simulink model "sf_tictacflow"  (Simulink 7.6)
settings: Solver=VariableStepDiscrete  StartTime=0.0  StopTime=inf  RelTol=1e-3
settings Model: Creator=The MathWorks Inc.  CovMetricSettings=dcmtr  ExtModeTrigMode=oneshot  ExtModeArmWhenConnect=off  ExtModeAutoUpdateStatusClock=off
settings DataIOCC: LimitDataPoints=off  SaveOutput=off  SaveTime=off  SignalLoggingName=sigsOut
settings OptimizationCC: BlockReduction=off  BooleanDataType=off  InlineInvariantSignals=on  InitFltsAndDblsToZero=on  EfficientMapNaN2IntZero=off  BufferReusableBoundary=off
settings DebuggingCC: SaveWithParameterizedLinksMsg=none  SignalResolutionControl=TryResolveAllWithWarning  SolverPrmCheckMsg=none  MultiTaskDSMMsg=warning  MultiTaskCondExecSysMsg=none  BusObjectLabelMismatch=none  StrictBusMsg=None
settings HardwareCC: TargetUnknown=on
settings SFSimCC: SFSimEcho=off  SimParseCustomCode=off
settings RTWCC: IncludeERTFirstTime=on
settings GRTTargetCC: TargetFcnLib=ansi_tfl_tmw.mat

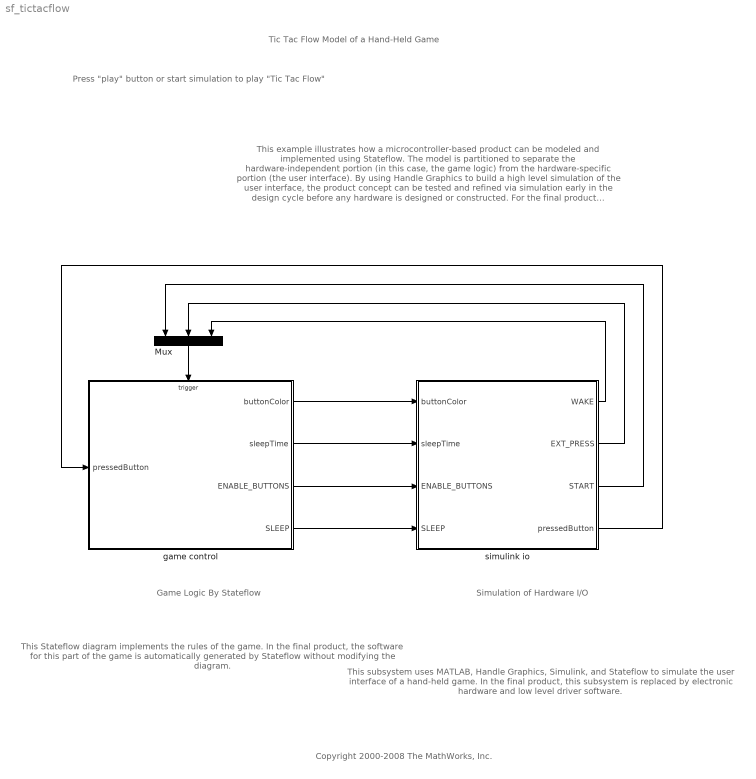
== system sf_tictacflow ==
  note: Press "play" button or start simulation to play "Tic Tac Flow"
  note: This Stateflow diagram implements
      | the rules of the game.
      |
      | In the final product, the software for this
      | part of the game is automatically generated
      |  by Stateflow without modifying the diagram.
  note: Game Logic By Stateflow
  note: This subsystem uses MATLAB, Handle
      | Graphics, Simulink, and Stateflow
      |  to simulate the user interface of a
      | hand-held game.
      |
      | In the final product, this subsystem is
      | replaced by electronic hardware and
      | low level driver software.
  note: This example illustrates how a microcontroller-based product can be modeled and implemented using Stateflow.
      |
      | The model is partitioned to separate the hardware-independent portion (in
      | this case, the game logic) from the hardware-specific portion (the user interface).
      | By using Handle Graphics to build a high level simulation of the user interface, the product concept can
      |  be tested and refined via simulation early in the design cycle before any hardware is designed or constructed.
      | For the final product implementation, the hardware-independent portion is implemented automatically
      |  by Stateflow, while the hardware-specific portion is replaced by actual hardware and low-level driver software.
  note: Tic Tac Flow
      | Model of a Hand-Held Game
  note: Simulation of Hardware I/O
  note: Copyright 2000-2008 The MathWorks, Inc.
  Mux : Mux  Inputs=3
  game control : Stateflow chart  TreatAsAtomicUnit=on
  simulink io : Subsystem  StopFcn=if ishandle(1.000000); delete(1.000000); end;
  wires:
  Mux/1 -> game control/Trigger
  game control/2(sleepTime) -> simulink io/2(sleepTime)
  game control/3(ENABLE_BUTTONS) -> simulink io/3(ENABLE_BUTTONS)
  game control/4(SLEEP) -> simulink io/4(SLEEP)
  game control/1(buttonColor) -> simulink io/1(buttonColor)
  simulink io/1(WAKE) -> Mux/3
  simulink io/2(EXT_PRESS) -> Mux/2
  simulink io/3(START) -> Mux/1
  simulink io/4(pressedButton) -> game control/1(pressedButton)

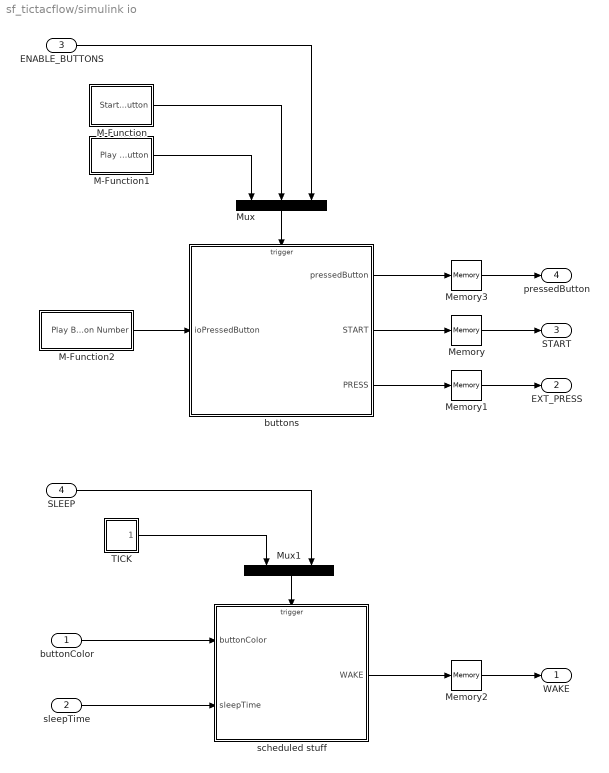
== system sf_tictacflow/simulink io ==
  buttonColor : Inport
  sleepTime : Inport  Port=2
  ENABLE_BUTTONS : Inport  Port=3
  SLEEP : Inport  Port=4
  M-Function : Subsystem
  M-Function1 : Subsystem
  M-Function2 : Subsystem
  Memory{,1..3} (4 alike) : Memory
  Mux : Mux  Inputs=3
  Mux1 : Mux  Inputs=2
  TICK : Subsystem  mask(Pulse Generator){period=1/60, duty=50, amplitude=1, start=0}
      mask prompts: period "Period (secs):"; duty "Duty cycle (% of period):"; start "Start time:"
      mask help: Pulse Generator
      mask Help: Pulse generator which ensures pulse transitions are hit. Provides a vector of pulses when the height is entered as a vector.  Unmask to see how it works.
      mask Display: plot(0,0,100,100,[95,90,90,75,75,60,60,45,45,30,30,15,15,5],[25,25,75,75,25,25,75,75,25,25,75,75,25,25]);
  buttons : Stateflow chart  TreatAsAtomicUnit=on
  scheduled stuff : Stateflow chart  TreatAsAtomicUnit=on
  WAKE : Outport
  EXT_PRESS : Outport  Port=2
  START : Outport  Port=3
  pressedButton : Outport  Port=4
  wires:
  Mux/1 -> buttons/Trigger
  Mux1/1 -> scheduled stuff/Trigger
  scheduled stuff/1(WAKE) -> Memory2/1
  Memory2/1 -> WAKE/1
  sleepTime/1 -> scheduled stuff/2(sleepTime)
  buttonColor/1 -> scheduled stuff/1(buttonColor)
  TICK/1(Out1) -> Mux1/1
  SLEEP/1 -> Mux1/2
  M-Function2/1(Play Button Number) -> buttons/1(ioPressedButton)
  M-Function1/1(Play Button) -> Mux/1
  M-Function/1(Start Button) -> Mux/2
  ENABLE_BUTTONS/1 -> Mux/3
  buttons/1(pressedButton) -> Memory3/1
  buttons/2(START) -> Memory/1
  Memory/1 -> START/1
  buttons/3(PRESS) -> Memory1/1
  Memory1/1 -> EXT_PRESS/1
  Memory3/1 -> pressedButton/1

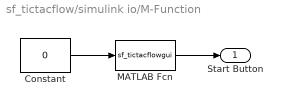
== system sf_tictacflow/simulink io/M-Function ==
  Constant : Constant  Value=0
  MATLAB Fcn : MATLABFcn  MATLABFcn=sf_tictacflowgui
  Start Button : Outport
  wires:
  Constant/1 -> MATLAB Fcn/1
  MATLAB Fcn/1 -> Start Button/1

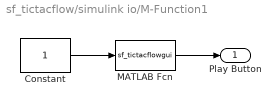
== system sf_tictacflow/simulink io/M-Function1 ==
  Constant : Constant
  MATLAB Fcn : MATLABFcn  MATLABFcn=sf_tictacflowgui
  Play Button : Outport
  wires:
  MATLAB Fcn/1 -> Play Button/1
  Constant/1 -> MATLAB Fcn/1

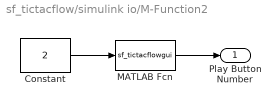
== system sf_tictacflow/simulink io/M-Function2 ==
  Constant : Constant  Value=2
  MATLAB Fcn : MATLABFcn  MATLABFcn=sf_tictacflowgui
  Play Button Number : Outport
  wires:
  Constant/1 -> MATLAB Fcn/1
  MATLAB Fcn/1 -> Play Button Number/1

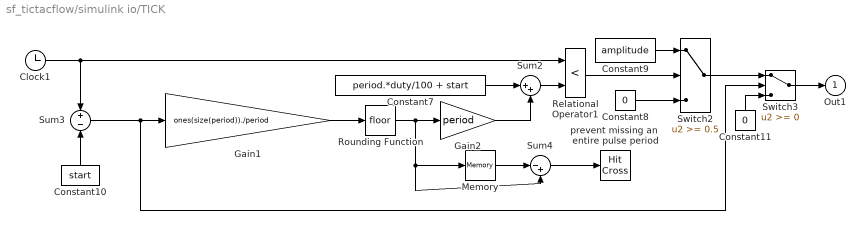
== system sf_tictacflow/simulink io/TICK ==
  Clock1 : Clock
      settings: Decimation=10
  Constant10 : Constant  Value=start
  Constant11 : Constant  Value=0
  Constant7 : Constant  Value=period.*duty/100 + start
  Constant8 : Constant  Value=0
  Constant9 : Constant  Value=amplitude
  Gain1 : Gain  Gain=ones(size(period))./period  SaturateOnIntegerOverflow=on  OutDataTypeStr=Inherit: Same as input  ParamDataTypeStr=Inherit: Same as input
  Gain2 : Gain  Gain=period  SaturateOnIntegerOverflow=on  OutDataTypeStr=Inherit: Same as input  ParamDataTypeStr=Inherit: Same as input
  Memory : Memory
  Relational Operator1 : RelationalOperator  Operator=<  InputSameDT=on
  Rounding Function : Rounding
  Sum2 : Sum  Inputs=|++  SaturateOnIntegerOverflow=on  InputSameDT=on  OutDataTypeStr=Inherit: Same as first input
  Sum3 : Sum  Inputs=+-  SaturateOnIntegerOverflow=on  InputSameDT=on  OutDataTypeStr=Inherit: Same as first input
  Sum4 : Sum  Inputs=|-+  SaturateOnIntegerOverflow=on  InputSameDT=on  OutDataTypeStr=Inherit: Same as first input
  Switch2 : Switch  Threshold=0.5  SaturateOnIntegerOverflow=on  InputSameDT=on
  Switch3 : Switch  SaturateOnIntegerOverflow=on  InputSameDT=on
  prevent missing an  entire pulse period : HitCross  HitCrossingOffset=1  ShowOutputPort=off
  Out1 : Outport
  wires:
  Memory/1 -> Sum4/1
  Sum4/1 -> prevent missing an  entire pulse period/1
  Switch2/1 -> Switch3/1
  Constant11/1 -> Switch3/3
  Constant9/1 -> Switch2/1
  Constant8/1 -> Switch2/3
  Relational Operator1/1 -> Switch2/2
  Switch3/1 -> Out1/1
  Rounding Function/1 -> Gain2/1, Memory/1, Sum4/2
  Gain2/1 -> Sum2/2
  Constant7/1 -> Sum2/1
  Gain1/1 -> Rounding Function/1
  Sum2/1 -> Relational Operator1/2
  Clock1/1 -> Sum3/1, Relational Operator1/1
  Sum3/1 -> Switch3/2, Gain1/1
  Constant10/1 -> Sum3/2

== stateflow chart game control ==
  settings: executeAtInitialization=1
  state button_7 [parallel]
    settings: executionOrder=1
    state enabled
      buttonColor[thisButton] = DARK;
    state active
      state green
        buttonColor[thisButton] = GREEN;
        TURN;
      state red
        buttonColor[thisButton] = RED;
        TURN;
      (junction 82) -> button_7.active.green [order 1] : [in(turn.green)]
      (junction 82) -> button_7.active.red [order 2]
    state disabled
    button_7.active.green -> button_7.disabled : GAME_OVER [in(turn.red)]
        | {buttonColor[thisButton] = DIM_GREEN; }
    button_7.enabled -> button_7.disabled [order 1] : GAME_OVER
    button_7 -> (junction 86) : START
    button_7.active -> button_7.enabled : at(7,TURN)
    (junction 86) -> button_7.enabled
    (default) -> (junction 86)
    button_7.enabled -> (junction 82) [order 2] : PRESS
    button_7.active.red -> button_7.disabled : GAME_OVER [in(turn.green)]
        | {buttonColor[thisButton] = DIM_RED; }
  state button_0 [parallel]
    settings: executionOrder=2
    state disabled
    state enabled
      buttonColor[thisButton] = DARK;
    state active
      state red
        buttonColor[thisButton] = RED;
        TURN;
      state green
        buttonColor[thisButton] = GREEN;
        TURN;
      (junction 105) -> button_0.active.red [order 2]
      (junction 105) -> button_0.active.green [order 1] : [in(turn.green)]
    button_0 -> (junction 104) : START
    (default) -> (junction 104)
    (junction 104) -> button_0.enabled
    button_0.enabled -> button_0.disabled [order 1] : GAME_OVER
    button_0.active.red -> button_0.disabled : GAME_OVER [in(turn.green)]
        | {buttonColor[thisButton] = DIM_RED; }
    button_0.active.green -> button_0.disabled : GAME_OVER [in(turn.red)]
        | {buttonColor[thisButton] = DIM_GREEN; }
    button_0.active -> button_0.enabled : at(7,TURN)
    button_0.enabled -> (junction 105) [order 2] : PRESS
  state button_5 [parallel]
    settings: executionOrder=3
    state disabled
    state enabled
      buttonColor[thisButton] = DARK;
    state active
      state red
        buttonColor[thisButton] = RED;
        TURN;
      state green
        buttonColor[thisButton] = GREEN;
        TURN;
      (junction 107) -> button_5.active.red [order 2]
      (junction 107) -> button_5.active.green [order 1] : [in(turn.green)]
    button_5 -> (junction 106) : START
    (default) -> (junction 106)
    (junction 106) -> button_5.enabled
    button_5.enabled -> button_5.disabled [order 1] : GAME_OVER
    button_5.active.red -> button_5.disabled : GAME_OVER [in(turn.green)]
        | {buttonColor[thisButton] = DIM_RED; }
    button_5.active.green -> button_5.disabled : GAME_OVER [in(turn.red)]
        | {buttonColor[thisButton] = DIM_GREEN; }
    button_5.active -> button_5.enabled : at(7,TURN)
    button_5.enabled -> (junction 107) [order 2] : PRESS
  state button_6 [parallel]
    settings: executionOrder=6
    state disabled
    state enabled
      buttonColor[thisButton] = DARK;
    state active
      state red
        buttonColor[thisButton] = RED;
        TURN;
      state green
        buttonColor[thisButton] = GREEN;
        TURN;
      (junction 109) -> button_6.active.red [order 2]
      (junction 109) -> button_6.active.green [order 1] : [in(turn.green)]
    button_6 -> (junction 108) : START
    (default) -> (junction 108)
    (junction 108) -> button_6.enabled
    button_6.enabled -> button_6.disabled [order 1] : GAME_OVER
    button_6.active.red -> button_6.disabled : GAME_OVER [in(turn.green)]
        | {buttonColor[thisButton] = DIM_RED; }
    button_6.active.green -> button_6.disabled : GAME_OVER [in(turn.red)]
        | {buttonColor[thisButton] = DIM_GREEN; }
    button_6.active -> button_6.enabled : at(7,TURN)
    button_6.enabled -> (junction 109) [order 2] : PRESS
  state button_4 [parallel]
    settings: executionOrder=5
    state disabled
    state enabled
      buttonColor[thisButton] = DARK;
    state active
      state red
        buttonColor[thisButton] = RED;
        TURN;
      state green
        buttonColor[thisButton] = GREEN;
        TURN;
      (junction 111) -> button_4.active.red [order 2]
      (junction 111) -> button_4.active.green [order 1] : [in(turn.green)]
    button_4 -> (junction 110) : START
    (default) -> (junction 110)
    (junction 110) -> button_4.enabled
    button_4.enabled -> button_4.disabled [order 1] : GAME_OVER
    button_4.active.red -> button_4.disabled : GAME_OVER [in(turn.green)]
        | {buttonColor[thisButton] = DIM_RED; }
    button_4.active.green -> button_4.disabled : GAME_OVER [in(turn.red)]
        | {buttonColor[thisButton] = DIM_GREEN; }
    button_4.active -> button_4.enabled : at(7,TURN)
    button_4.enabled -> (junction 111) [order 2] : PRESS
  state button_2 [parallel]
    settings: executionOrder=4
    state disabled
    state enabled
      buttonColor[thisButton] = DARK;
    state active
      state red
        buttonColor[thisButton] = RED;
        TURN;
      state green
        buttonColor[thisButton] = GREEN;
        TURN;
      (junction 113) -> button_2.active.red [order 2]
      (junction 113) -> button_2.active.green [order 1] : [in(turn.green)]
    button_2 -> (junction 112) : START
    (default) -> (junction 112)
    (junction 112) -> button_2.enabled
    button_2.enabled -> button_2.disabled [order 1] : GAME_OVER
    button_2.active.red -> button_2.disabled : GAME_OVER [in(turn.green)]
        | {buttonColor[thisButton] = DIM_RED; }
    button_2.active.green -> button_2.disabled : GAME_OVER [in(turn.red)]
        | {buttonColor[thisButton] = DIM_GREEN; }
    button_2.active -> button_2.enabled : at(7,TURN)
    button_2.enabled -> (junction 113) [order 2] : PRESS
  state button_1 [parallel]
    settings: executionOrder=9
    state disabled
    state enabled
      buttonColor[thisButton] = DARK;
    state active
      state red
        buttonColor[thisButton] = RED;
        TURN;
      state green
        buttonColor[thisButton] = GREEN;
        TURN;
      (junction 115) -> button_1.active.red [order 2]
      (junction 115) -> button_1.active.green [order 1] : [in(turn.green)]
    button_1 -> (junction 114) : START
    (default) -> (junction 114)
    (junction 114) -> button_1.enabled
    button_1.enabled -> button_1.disabled [order 1] : GAME_OVER
    button_1.active.red -> button_1.disabled : GAME_OVER [in(turn.green)]
        | {buttonColor[thisButton] = DIM_RED; }
    button_1.active.green -> button_1.disabled : GAME_OVER [in(turn.red)]
        | {buttonColor[thisButton] = DIM_GREEN; }
    button_1.active -> button_1.enabled : at(7,TURN)
    button_1.enabled -> (junction 115) [order 2] : PRESS
  state button_8 [parallel]
    settings: executionOrder=8
    state disabled
    state enabled
      buttonColor[thisButton] = DARK;
    state active
      state red
        buttonColor[thisButton] = RED;
        TURN;
      state green
        buttonColor[thisButton] = GREEN;
        TURN;
      (junction 117) -> button_8.active.red [order 2]
      (junction 117) -> button_8.active.green [order 1] : [in(turn.green)]
    button_8 -> (junction 116) : START
    (default) -> (junction 116)
    (junction 116) -> button_8.enabled
    button_8.enabled -> button_8.disabled [order 1] : GAME_OVER
    button_8.active.red -> button_8.disabled : GAME_OVER [in(turn.green)]
        | {buttonColor[thisButton] = DIM_RED; }
    button_8.active.green -> button_8.disabled : GAME_OVER [in(turn.red)]
        | {buttonColor[thisButton] = DIM_GREEN; }
    button_8.active -> button_8.enabled : at(7,TURN)
    button_8.enabled -> (junction 117) [order 2] : PRESS
  state button_3 [parallel]
    settings: executionOrder=7
    state disabled
    state enabled
      buttonColor[thisButton] = DARK;
    state active
      state red
        buttonColor[thisButton] = RED;
        TURN;
      state green
        buttonColor[thisButton] = GREEN;
        TURN;
      (junction 119) -> button_3.active.red [order 2]
      (junction 119) -> button_3.active.green [order 1] : [in(turn.green)]
    button_3 -> (junction 118) : START
    (default) -> (junction 118)
    (junction 118) -> button_3.enabled
    button_3.enabled -> button_3.disabled [order 1] : GAME_OVER
    button_3.active.red -> button_3.disabled : GAME_OVER [in(turn.green)]
        | {buttonColor[thisButton] = DIM_RED; }
    button_3.active.green -> button_3.disabled : GAME_OVER [in(turn.red)]
        | {buttonColor[thisButton] = DIM_GREEN; }
    button_3.active -> button_3.enabled : at(7,TURN)
    button_3.enabled -> (junction 119) [order 2] : PRESS
  state turn [parallel]
    settings: executionOrder=10
    state yes = make_move_if_available(move) [function]
      (junction 89) -> (junction 77)
      (junction 97) -> (junction 88) [order 2]
      (junction 88) -> (junction 78) [order 1] : [ move == 8 && in(button_8.enabled)] { shift_game_state(move); send(PRESS,button_8);}
      (junction 99) -> (junction 97) [order 2]
      (default) -> (junction 70)
      (junction 98) -> (junction 96)
      (junction 88) -> (junction 85) [order 2] : { yes = 0; }
      (junction 97) -> (junction 96) [order 1] : [ move == 7 && in(button_7.enabled)] { shift_game_state(move); send(PRESS,button_7);}
      (junction 70) -> (junction 80) [order 1] : [ move == 0 && in(button_0.enabled)] { shift_game_state(move); send(PRESS,button_0);}
      (junction 102) -> (junction 100)
      (junction 77) -> (junction 102)
      (junction 72) -> (junction 89)
      (junction 103) -> (junction 102) [order 1] : [ move == 4 && in(button_4.enabled)] { shift_game_state(move); send(PRESS,button_4);}
      (junction 80) -> (junction 72)
      (junction 78) -> (junction 92) : { yes = 1; }
      (junction 101) -> (junction 100) [order 1] : [ move == 5 && in(button_5.enabled)] { shift_game_state(move); send(PRESS,button_5);}
      (junction 70) -> (junction 68) [order 2]
      (junction 100) -> (junction 98)
      (junction 68) -> (junction 72) [order 1] : [ move == 1 && in(button_1.enabled)] { shift_game_state(move); send(PRESS,button_1);}
      (junction 90) -> (junction 89) [order 1] : [ move == 2 && in(button_2.enabled)] { shift_game_state(move); send(PRESS,button_2);}
      (junction 68) -> (junction 90) [order 2]
      (junction 76) -> (junction 77) [order 1] : [ move == 3 && in(button_3.enabled)] { shift_game_state(move); send(PRESS,button_3);}
      (junction 90) -> (junction 76) [order 2]
      (junction 76) -> (junction 103) [order 2]
      (junction 99) -> (junction 98) [order 1] : [ move == 6 && in(button_6.enabled)] { shift_game_state(move); send(PRESS,button_6);}
      (junction 103) -> (junction 101) [order 2]
      (junction 101) -> (junction 99) [order 2]
      (junction 96) -> (junction 78)
    state shift_game_state(magicNumber) [function]
      (default) -> (junction 87) : {
          |   gameState[5] = gameState[4];
          |   gameState[4] = gameState[3];
          |   gameState[3] = gameState[2];
          |   gameState[2] = gameState[1];
          |   gameState[1] = gameState[0];
          |   gameState[0] = magicNumber;
          | }
    state red
      buttonColor[9] = RED;
      ENABLE_BUTTONS;
    state yes = is_a_winner() [function]
      (default) -> (junction 81) : { yes =((gameState[0] + gameState[2] + gameState[4]) == 12); }
    state game_over
    state green
      buttonColor[9] = GREEN;
      state awakened
        choose_move();
      state two_player
        ENABLE_BUTTONS;
      state sleeping
        sleepTime = 255;
        SLEEP;
      sleeping -> awakened : WAKE
      (junction 120) -> two_player [order 1] : [TWO_PLAYER]
      (junction 120) -> sleeping [order 2]
      (default) -> (junction 120)
    state move = choose_move() [function]
      (junction 73) -> (junction 91) [order 1] : [ make_move_if_available(move) ]
      (junction 95) -> (junction 94)
      (default) -> (junction 79) : /* try to win on this move */
          | { move = 12 - gameState[1] - gameState[3]; }
      (junction 79) -> (junction 74) [order 1] : [ make_move_if_available(move) ]
      (junction 73) -> (junction 83) [order 2] : /* else make a random  move */
          | { move = seed; }
      (junction 94) -> (junction 83)
      (junction 83) -> (junction 75) : {
          |   /* simple linear congruential
          |      pseudo-random sequence:
          |      x = (5x + 3) mod 16 */
          |   move += move << 2;
          |   move += 3;
          |   move &= 0xf;
          | }
      (junction 75) -> (junction 95) [order 1] : [!make_move_if_available(move)]
      (junction 75) -> (junction 69) [order 2] : { seed = move; }
      (junction 79) -> (junction 73) [order 2] : /* else try to block opponent from winning next move */
          | { move = 12 - gameState[0] - gameState[2]; }
    (junction 93) -> game_over [order 1] : [is_a_winner()] {GAME_OVER;}
    (junction 84) -> turn.green [order 2]
    turn.red -> (junction 84) : TURN
    (junction 93) -> turn.red [order 2]
    (junction 84) -> game_over [order 1] : [is_a_winner()] {GAME_OVER; }
    turn -> (junction 71) [order 2] : START
    (default) -> (junction 71)
    (junction 71) -> turn.red : { gameState = 13; }
    turn.green -> (junction 93) : TURN
    turn -> (junction 121) [order 1] : EXT_PRESS
    (junction 121) -> (junction 122) [order 1] : [ make_move_if_available( pressedButton ) ]
    (junction 121) -> (junction 123) [order 2] : { ENABLE_BUTTONS; }
  data: move function_input int8; yes function_output boolean; magicNumber function_input uint8; thisButton constant uint8 =7; yes function_output boolean; sum temporary uint8; count temporary uint8; move function_output int8; thisButton constant uint8; thisButton constant uint8 =5; thisButton constant uint8 =6; thisButton constant uint8 =4; thisButton constant uint8 =2; thisButton constant uint8 =1; thisButton constant uint8 =8; thisButton constant uint8 =3; gameState local int8 size=9; seed local uint8 =13; RED constant uint8 =15; DIM_RED constant uint8 =8; GREEN constant uint8 =240; DIM_GREEN constant uint8 =128; DARK constant uint8; YELLOW constant uint8 =255; TWO_PLAYER constant boolean; buttonColor output uint8 size=10; sleepTime output uint8; pressedButton input uint8
  events: TURN local EITHER_EDGE_EVENT; GAME_OVER local EITHER_EDGE_EVENT; ENABLE_BUTTONS output EITHER_EDGE_EVENT; START input EITHER_EDGE_EVENT; EXT_PRESS input EITHER_EDGE_EVENT; PRESS local EITHER_EDGE_EVENT; SLEEP output EITHER_EDGE_EVENT; WAKE input EITHER_EDGE_EVENT

== stateflow chart simulink io/buttons ==
  settings: sampleTime=1  executeAtInitialization=1
  state io [parallel]
    en:
    figH = ml.sf_tictacflowgui('fig');
    ml.set(figH,'Pointer','arrow');
    /* note mapping between magic numbers and button location:
    buttonH[magic] = ml.play_button_magic(figH,location,magic);  */
    buttonH[0] = ml.sf_tictacflowgui('play_button',figH,1,0);
    buttonH[1] = ml.sf_tictacflowgui('play_button',figH,8,1);
    buttonH[2] = ml.sf_tictacflowgui('play_button',figH,3,2);
    buttonH[3] = ml.sf_tictacflowgui('play_button',figH,6,3);
    buttonH[4] = ml.sf_tictacflowgui('play_button',figH,4,4);
    buttonH[5] = ml.sf_tictacflowgui('play_button',figH,2,5);
    buttonH[6] = ml.sf_tictacflowgui('play_button',figH,5,6);
    buttonH[7] = ml.sf_tictacflowgui('play_button',figH,0,7);
    buttonH[8] = ml.sf_tictacflowgui('play_button',figH,7,8);
    startButtonH = ml.sf_tictacflowgui('start_button',figH);
    turnSignalH = ml.sf_tictacflowgui('turn_signal',figH);
    settings: executionOrder=1
    (junction 315) -> (junction 309) [order 2]
    (junction 313) -> (junction 311) [order 1] : IO_START
        | {
        |    pressedButton = 0;
        |    START;
        | }
    (junction 315) -> (junction 312) [order 1] : IO_PRESS
        | {
        |   ml.set(buttonH[0],'Enable','Off');
        |   ml.set(buttonH[1],'Enable','Off');
        |   ml.set(buttonH[2],'Enable','Off');
        |   ml.set(buttonH[3],'Enable','Off');
        |   ml.set(buttonH[4],'Enable','Off');
        |   ml.set(buttonH[5],'Enable','Off');
        |   ml.set(buttonH[6],'Enable','Off');
        |   ml.set(buttonH[7],'Enable','Off');
        |   ml.set(buttonH[8],'Enable','Off');
        |   pressedButton = ioPressedButton;
        |   PRESS;
        | }
    (junction 314) -> (junction 310) [order 1] : ENABLE_BUTTONS
        | {
        |   ml.set(buttonH[0],'Enable','On');
        |   ml.set(buttonH[1],'Enable','On');
        |   ml.set(buttonH[2],'Enable','On');
        |   ml.set(buttonH[3],'Enable','On');
        |   ml.set(buttonH[4],'Enable','On');
        |   ml.set(buttonH[5],'Enable','On');
        |   ml.set(buttonH[6],'Enable','On');
        |   ml.set(buttonH[7],'Enable','On');
        |   ml.set(buttonH[8],'Enable','On');
        | }
    io -> (junction 313)
    (junction 313) -> (junction 314) [order 2]
    (junction 314) -> (junction 315) [order 2]
  data: startButtonH local double; ioPressedButton input double; pressedButton output uint8
  events: IO_PRESS input EITHER_EDGE_EVENT; IO_START input EITHER_EDGE_EVENT; ENABLE_BUTTONS input EITHER_EDGE_EVENT; START output EITHER_EDGE_EVENT; PRESS output EITHER_EDGE_EVENT

== stateflow chart simulink io/scheduled stuff ==
  settings: sampleTime=1  executeAtInitialization=1
  state sleep [parallel]
    settings: executionOrder=3
    state asleep
      entry:
      ml.set(figH,'Pointer','watch');
      exit:
      ml.set(figH,'Pointer','arrow');
    state awake
    (default) -> awake
    asleep -> awake : after(sleepTime,TICK)
        | { WAKE; }
    awake -> asleep : SLEEP
  state stop [parallel]
    settings: executionOrder=1
    stop -> (junction 340)
    (default) -> (junction 340)
    (junction 340) -> (junction 339) : [ !ml.ishandle(figH) ]
        | { ml.set_param('sf_tictacflow','simulationcommand','stop'); }
  state update_LEDs [parallel]
    settings: executionOrder=2
    (junction 341) -> (junction 338) : TICK
        | [ml.ishandle(figH)]
        | {
        |   ml.sf_tictacflowgui('set_button_color',buttonH[0],buttonColor[0]);
        |   ml.sf_tictacflowgui('set_button_color',buttonH[1],buttonColor[1]);
        |   ml.sf_tictacflowgui('set_button_color',buttonH[2],buttonColor[2]);
        |   ml.sf_tictacflowgui('set_button_color',buttonH[3],buttonColor[3]);
        |   ml.sf_tictacflowgui('set_button_color',buttonH[4],buttonColor[4]);
        |   ml.sf_tictacflowgui('set_button_color',buttonH[5],buttonColor[5]);
        |   ml.sf_tictacflowgui('set_button_color',buttonH[6],buttonColor[6]);
        |   ml.sf_tictacflowgui('set_button_color',buttonH[7],buttonColor[7]);
        |   ml.sf_tictacflowgui('set_button_color',buttonH[8],buttonColor[8]);
        |   ml.sf_tictacflowgui('set_button_color',turnSignalH,buttonColor[9]);
        | }
    update_LEDs -> (junction 341)
    (default) -> (junction 341)
  data: oldPtr local double; buttonColor input uint8 size=10; sleepTime input uint8
  events: TICK input EITHER_EDGE_EVENT; SLEEP input EITHER_EDGE_EVENT; WAKE output EITHER_EDGE_EVENT
